simulink subsystem "VL53X_multipleSensor"  (R2023b)
settings: Solver=VariableStepAuto  StartTime=0.0  StopTime=10.0  RelTol=1e-3
settings Model: Creator=m4ttn  LastModifiedBy=m4ttn

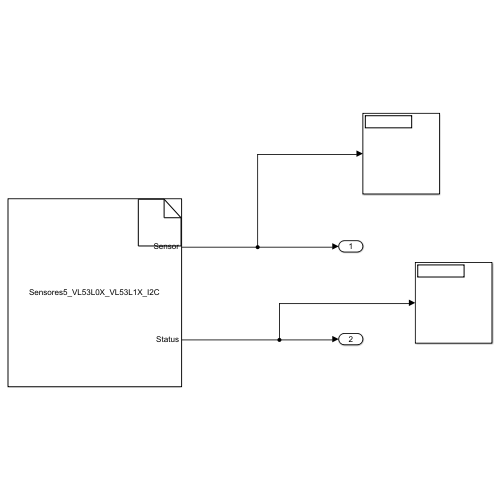
[thumbnail: Simulink's stored preview of the top-level diagram]
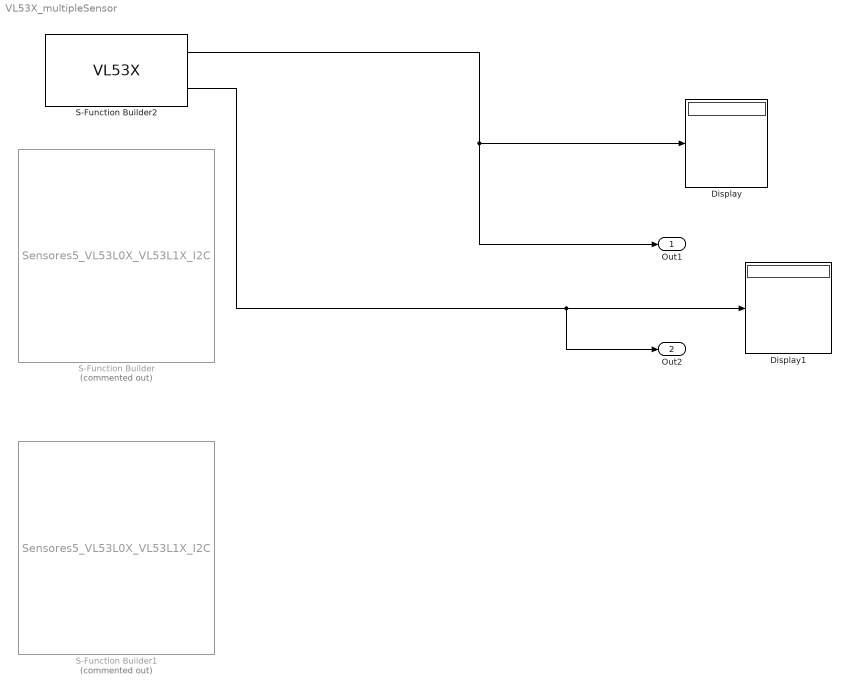
== system VL53X_multipleSensor ==
  Display : Display
  Display1 : Display
  S-Function Builder : S-Function  Commented=on  InitFcn=try, set_param(gcb,'FunctionName','Sensores5_VL53L0X_VL53L1X_I2C'), end  FunctionName=Sensores5_VL53L0X_VL53L1X_I2C  SFunctionModules=VL53L0X_VL53L1X_I2C_wrapper.cpp  SFunctionDeploymentMode=off  EnableBusSupport=off  mask(S-Function Builder){}
      mask help: Simulink:masks:SFunctionBuilder_MD
      mask init:
      | val = [[.9  0.75 0.75 1 1 .9 .9 1]',[1 1 0.75 0.75 .9 .9 1 .9]'];try , sys = get_param(gcb,'SfunBuilderFcnName');if isempty(sys), sys = get_param(gcb,'FunctionName'); end,catch, sys = get_param(gcb,'FunctionName'); end
      settings: CopyFcn=set_param(gcbh,'LinkStatus','none')  PreSaveFcn=try, set_param(gcb,'FunctionName','Sensores5_VL53L0X_VL53L1X_I2C'), end  OpenFcn=sfunctionwizard(gcbh)
      mask Display:
      | plot(val(:,1),val(:,2))
      | disp(sys)
      | port_label('output',1,'Sensor')
      | port_label('output',2,'Status')
  S-Function Builder1 : S-Function  Commented=on  InitFcn=try, set_param(gcb,'FunctionName','Sensores5_VL53L0X_VL53L1X_I2C'), end  FunctionName=Sensores5_VL53L0X_VL53L1X_I2C  SFunctionModules=Sensores5_VL53L0X_VL53L1X_I2C_wrapper.cpp  SFunctionDeploymentMode=off  EnableBusSupport=off  mask(S-Function Builder){}
      mask help: Simulink:masks:SFunctionBuilder_MD
      mask init: same as VL53X_multipleSensor/S-Function Builder
      settings: CopyFcn=set_param(gcbh,'LinkStatus','none')  PreSaveFcn=try, set_param(gcb,'FunctionName','Sensores5_VL53L0X_VL53L1X_I2C'), end  OpenFcn=sfunctionwizard(gcbh)
      mask Display:
      | plot(val(:,1),val(:,2))
      | disp(sys)
      | port_label('output',1,'Sensor')
      | port_label('output',2,'Status')
  S-Function Builder2 : S-Function  FunctionName=VL53X  SFunctionModules=VL53X_wrapper.cpp  SFunctionDeploymentMode=off  EnableBusSupport=off  mask(S-Function Builder){}
      mask help: Simulink:masks:SFunctionBuilder_MD
      mask init: same as VL53X_multipleSensor/S-Function Builder
      settings: CopyFcn=set_param(gcbh,'LinkStatus','none')  OpenFcn=sfunctionwizard(gcbh)
      mask Display:
      | plot(val(:,1),val(:,2))
      | disp(sys)
      | port_label('output',1,'Sensor')
      | port_label('output',2,'Status')
  Out1 : Outport
  Out2 : Outport  Port=2
  wires:
  S-Function Builder2/1 -> Display/1, Out1/1
  S-Function Builder2/2 -> Display1/1, Out2/1
